simulink model "Erro_RP"  (R2016a)
settings: Solver=VariableStepAuto  StartTime=0.0  StopTime=50  RelTol=1e-3
libraries: simulink x2
settings Model: Creator=andre  LastModifiedBy=andre

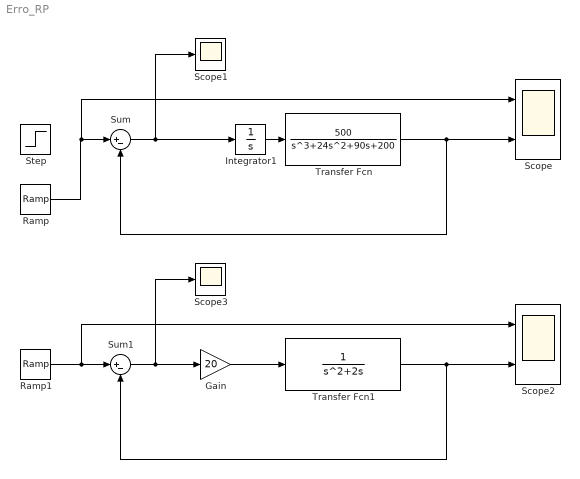
== system Erro_RP ==
  Gain : Gain  Gain=20
  Integrator1 : Integrator
  Ramp : simulink/Sources/Ramp  slope=70  start=0  X0=0
  Ramp1 : simulink/Sources/Ramp  slope=1  start=0  X0=0
  Scope : Scope  NumInputPorts=2
  Scope1 : Scope
  Scope2 : Scope  NumInputPorts=2
  Scope3 : Scope
  Step : Step  Time=0  After=40  SampleTime=0
  Sum : Sum  Inputs=|+-
  Sum1 : Sum  Inputs=|+-
  Transfer Fcn : TransferFcn  Numerator=[0 500]  Denominator=[1 24 90 200]
  Transfer Fcn1 : TransferFcn  Denominator=[1 2 0]
  wires:
  Transfer Fcn/1 -> Scope/2, Sum/2
  Sum/1 -> Integrator1/1, Scope1/1
  Ramp/1 -> Scope/1, Sum/1
  Integrator1/1 -> Transfer Fcn/1
  Transfer Fcn1/1 -> Scope2/2, Sum1/2
  Ramp1/1 -> Scope2/1, Sum1/1
  Sum1/1 -> Gain/1, Scope3/1
  Gain/1 -> Transfer Fcn1/1
